simulink model "Test"  (R2019a)
settings: Solver=VariableStepAuto  StartTime=0.0  StopTime=15  RelTol=1e-3
values from neighbouring files (symbols this model uses):
  a = [a2(1);a1(1);a2(2);a1(2);a2(3)]    [ID.m]
  b = Bluetooth('u_t_chan',1)    [Data.m]    (also in ID.m = [b2(1);b2(2);b1(1);b1(2);b2(3)])
undefined symbols (not defined in the file or in its folder): DiscIntNeverNeededParam
libraries: simulink x2
settings Model: Creator=ray  LastModifiedBy=USER
settings DebuggingCC: AlgebraicLoopMsg=none

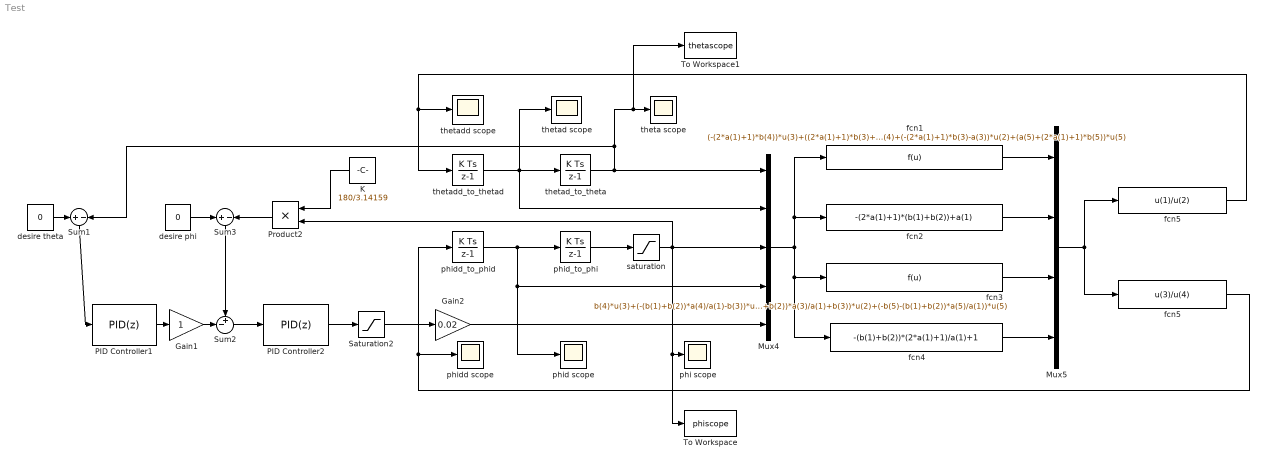
== system Test ==
  Gain1 : Gain
  Gain2 : Gain  Gain=0.02
  K : Constant  Value=180/3.14159  SampleTime=0.01
  Mux4 : Mux  Inputs=5
  Mux5 : Mux
  PID Controller1 : simulink/Continuous/PID Controller  Controller=PID  Form=Parallel  TimeDomain=Discrete-time  SampleTime=0.001  IntegratorMethod=Forward Euler  FilterMethod=Forward Euler  ControllerParametersSource=internal  P=0.9  I=0.01  D=-0.133  UseFilter=on  N=3.92484448633135  TunerSelectOption=Transfer Function Based (PID Tuner App)  InitialConditionSource=internal  InitialConditionForIntegrator=0  InitialConditionForFilter=0  DifferentiatorICPrevScaledInput=0  ExternalReset=none  TrackingMode=off  Kt=1  LimitOutput=off  UpperSaturationLimit=inf  LowerSaturationLimit=-inf  LinearizeAsGain=on  AntiWindupMode=none  Kb=1  POutMin=[]  POutMax=[]  IOutMin=[]  IOutMax=[]  DOutMin=[]  DOutMax=[]  NOutMin=[]  NOutMax=[]  SumOutMin=[]  SumOutMax=[]  SaturationOutMin=[]  SaturationOutMax=[]  PParamMin=[]  PParamMax=[]  IParamMin=[]  IParamMax=[]  DParamMin=[]  DParamMax=[]  NParamMin=[]  NParamMax=[]  KbParamMin=[]  KbParamMax=[]  KtParamMin=[]  KtParamMax=[]  KbOutMin=[]  KbOutMax=[]  KtOutMin=[]  KtOutMax=[]  IntegratorOutMin=[]  IntegratorOutMax=[]  FilterOutMin=[]  FilterOutMax=[]  SumI1OutMin=[]  SumI1OutMax=[]  SumI2OutMin=[]  SumI2OutMax=[]  SumI3OutMin=[]  SumI3OutMax=[]  SumI4OutMin=[]  SumI4OutMax=[]  SumDOutMin=[]  SumDOutMax=[]  DifferentiatorOutMin=[]  DifferentiatorOutMax=[]  FilterDiffOutCoefMin=[]  FilterDiffOutCoefMax=[]  ReciprocalOutMin=[]  ReciprocalOutMax=[]  SumDenOutMin=[]  SumDenOutMax=[]  SumNumOutMin=[]  SumNumOutMax=[]  DivideOutMin=[]  DivideOutMax=[]  IntegratorContinuousStateAttributes=''  IntegratorStateMustResolveToSignalObject=off  IntegratorRTWStateStorageClass=Auto  FilterContinuousStateAttributes=''  FilterStateMustResolveToSignalObject=off  FilterRTWStateStorageClass=Auto  ParallelPVariant=InternalParameters  IdealPVariant=Disabled  IVariant=InternalParameters  DVariant=InternalParameters  IntegratorVariant=Discrete  SatVariant=Disabled  AWVariant=Passthrough  PCopyVariant=Disabled  TRVariant=Disabled  FdbkBlocksVariant=Forward  IdealPFdbkVariant=Disabled  SatFdbkVariant=Disabled  DerivativeFilterVariant=ForwardEulerFilter  NVariant=InternalParameters  NCopyVariant=Disabled  FilterICVariant=InternalICsFilter  IntegratorICVariant=InternalICs  ExternalResetVariant=Disabled  TRSumVariant=Passthrough  SumFdbkVariant=Disabled  SumVariant=Sum_PID
  PID Controller2 : simulink/Continuous/PID Controller  Controller=PID  Form=Parallel  TimeDomain=Discrete-time  SampleTime=0.001  IntegratorMethod=Forward Euler  FilterMethod=Forward Euler  ControllerParametersSource=internal  P=10  I=100  D=1  UseFilter=on  N=100  TunerSelectOption=Transfer Function Based (PID Tuner App)  InitialConditionSource=internal  InitialConditionForIntegrator=0  InitialConditionForFilter=0  DifferentiatorICPrevScaledInput=0  ExternalReset=none  TrackingMode=off  Kt=1  LimitOutput=off  UpperSaturationLimit=inf  LowerSaturationLimit=-inf  LinearizeAsGain=on  AntiWindupMode=none  Kb=1  POutMin=[]  POutMax=[]  IOutMin=[]  IOutMax=[]  DOutMin=[]  DOutMax=[]  NOutMin=[]  NOutMax=[]  SumOutMin=[]  SumOutMax=[]  SaturationOutMin=[]  SaturationOutMax=[]  PParamMin=[]  PParamMax=[]  IParamMin=[]  IParamMax=[]  DParamMin=[]  DParamMax=[]  NParamMin=[]  NParamMax=[]  KbParamMin=[]  KbParamMax=[]  KtParamMin=[]  KtParamMax=[]  KbOutMin=[]  KbOutMax=[]  KtOutMin=[]  KtOutMax=[]  IntegratorOutMin=[]  IntegratorOutMax=[]  FilterOutMin=[]  FilterOutMax=[]  SumI1OutMin=[]  SumI1OutMax=[]  SumI2OutMin=[]  SumI2OutMax=[]  SumI3OutMin=[]  SumI3OutMax=[]  SumI4OutMin=[]  SumI4OutMax=[]  SumDOutMin=[]  SumDOutMax=[]  DifferentiatorOutMin=[]  DifferentiatorOutMax=[]  FilterDiffOutCoefMin=[]  FilterDiffOutCoefMax=[]  ReciprocalOutMin=[]  ReciprocalOutMax=[]  SumDenOutMin=[]  SumDenOutMax=[]  SumNumOutMin=[]  SumNumOutMax=[]  DivideOutMin=[]  DivideOutMax=[]  IntegratorContinuousStateAttributes=''  IntegratorStateMustResolveToSignalObject=off  IntegratorRTWStateStorageClass=Auto  FilterContinuousStateAttributes=''  FilterStateMustResolveToSignalObject=off  FilterRTWStateStorageClass=Auto  ParallelPVariant=InternalParameters  IdealPVariant=Disabled  IVariant=InternalParameters  DVariant=InternalParameters  IntegratorVariant=Discrete  SatVariant=Disabled  AWVariant=Passthrough  PCopyVariant=Disabled  TRVariant=Disabled  FdbkBlocksVariant=Forward  IdealPFdbkVariant=Disabled  SatFdbkVariant=Disabled  DerivativeFilterVariant=ForwardEulerFilter  NVariant=InternalParameters  NCopyVariant=Disabled  FilterICVariant=InternalICsFilter  IntegratorICVariant=InternalICs  ExternalResetVariant=Disabled  TRSumVariant=Passthrough  SumFdbkVariant=Disabled  SumVariant=Sum_PID
  Product2 : Product
  Saturation2 : Saturate  UpperLimit=255  LowerLimit=-255
  Sum1 : Sum  Inputs=+-
  Sum2 : Sum  Inputs=+-|
  Sum3 : Sum  Inputs=+-
  To Workspace : ToWorkspace  VariableName=phiscope  SaveFormat=Timeseries  SampleTime=-1
  To Workspace1 : ToWorkspace  VariableName=thetascope  SaveFormat=Timeseries  SampleTime=-1
  desire phi : Constant  Value=0  SampleTime=0.01
  desire theta : Constant  Value=0  SampleTime=0.01
  fcn1 : Fcn  Expr=(-(2*a(1)+1)*b(4))*u(3)+((2*a(1)+1)*b(3)+a(4))*u(4)+(-(2*a(1)+1)*b(3)-a(3))*u(2)+(a(5)+(2*a(1)+1)*b(5))*u(5)
  fcn2 : Fcn  Expr=-(2*a(1)+1)*(b(1)+b(2))+a(1)
  fcn3 : Fcn  Expr=b(4)*u(3)+(-(b(1)+b(2))*a(4)/a(1)-b(3))*u(4)+((b(1)+b(2))*a(3)/a(1)+b(3))*u(2)+(-b(5)-(b(1)+b(2))*a(5)/a(1))*u(5)
  fcn4 : Fcn  Expr=-(b(1)+b(2))*(2*a(1)+1)/a(1)+1
  fcn5 : Fcn  Expr=u(3)/u(4)
  "fcn5 " : Fcn  Expr=u(1)/u(2)
  phi scope : Scope
  phid scope : Scope
  "phid_to_phi " : DiscreteIntegrator  SampleTime=0.001  ICPrevOutput=DiscIntNeverNeededParam  ICPrevScaledInput=DiscIntNeverNeededParam
  phidd scope : Scope
  phidd_to_phid : DiscreteIntegrator  SampleTime=0.001  ICPrevOutput=DiscIntNeverNeededParam  ICPrevScaledInput=DiscIntNeverNeededParam
  saturation : Saturate  UpperLimit=1.6  LowerLimit=-1.6
  "theta scope " : Scope
  thetad scope : Scope
  thetad_to_theta : DiscreteIntegrator  SampleTime=0.001  ICPrevOutput=DiscIntNeverNeededParam  ICPrevScaledInput=DiscIntNeverNeededParam
  thetadd scope : Scope
  thetadd_to_thetad : DiscreteIntegrator  SampleTime=0.001  ICPrevOutput=DiscIntNeverNeededParam  ICPrevScaledInput=DiscIntNeverNeededParam
  wires:
  "fcn5 "/1 -> thetadd scope/1, thetadd_to_thetad/1
  PID Controller2/1 -> Saturation2/1
  Product2/1 -> Sum3/2
  fcn4/1 -> Mux5/4
  K/1 -> Product2/1
  Mux5/1 -> fcn5/1, "fcn5 "/1
  desire phi/1 -> Sum3/1
  fcn1/1 -> Mux5/1
  fcn2/1 -> Mux5/2
  thetadd_to_thetad/1 -> thetad_to_theta/1, Mux4/2, thetad scope/1
  phidd_to_phid/1 -> "phid_to_phi "/1, Mux4/4, phid scope/1
  Mux4/1 -> fcn1/1, fcn2/1, fcn4/1, fcn3/1
  saturation/1 -> To Workspace/1, phi scope/1, Mux4/3, Product2/2
  "phid_to_phi "/1 -> saturation/1
  fcn3/1 -> Mux5/3
  thetad_to_theta/1 -> Mux4/1, Sum1/2, To Workspace1/1, "theta scope "/1
  fcn5/1 -> phidd scope/1, phidd_to_phid/1
  Saturation2/1 -> Gain2/1
  Gain2/1 -> Mux4/5
  desire theta/1 -> Sum1/1
  Sum1/1 -> PID Controller1/1
  Sum3/1 -> Sum2/1
  Sum2/1 -> PID Controller2/1
  PID Controller1/1 -> Gain1/1
  Gain1/1 -> Sum2/2
